simulink model "complex_with_subsystems"  (Simulink 8.0)
settings: Solver=ode45  StartTime=0.0  StopTime=10.0  MaxStep=0.1  RelTol=1e-3
settings Model: Creator=rstarr  LastModifiedBy=rstarr

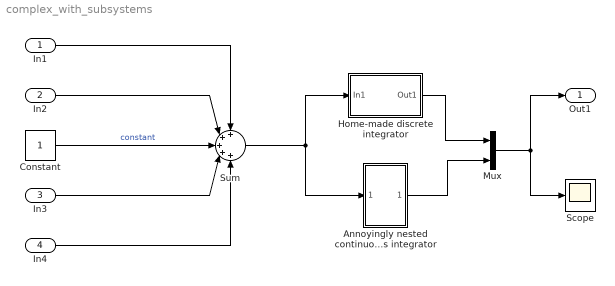
== system complex_with_subsystems ==
  In1 : Inport
  In2 : Inport  Port=2
  In3 : Inport  Port=3
  In4 : Inport  Port=4
  Annoyingly nested continuous integrator : Subsystem
  Constant : Constant
  Home-made discrete integrator : Subsystem
  Mux : Mux  Inputs=2
  Scope : Scope
  Sum : Sum  Inputs=+++++
  Out1 : Outport
  wires:
  Constant/1 -> Sum/3  "constant"
  In2/1 -> Sum/2
  In3/1 -> Sum/4
  In1/1 -> Sum/1
  In4/1 -> Sum/5
  Sum/1 -> Annoyingly nested continuous integrator/1(In1), Home-made discrete integrator/1(In1)
  Mux/1 -> Out1/1, Scope/1
  Home-made discrete integrator/1(Out1) -> Mux/1
  Annoyingly nested continuous integrator/1(Out1) -> Mux/2

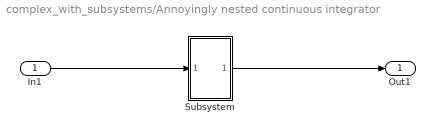
== system complex_with_subsystems/Annoyingly nested continuous integrator ==
  In1 : Inport
  Subsystem : Subsystem
  Out1 : Outport
  wires:
  In1/1 -> Subsystem/1(In1)
  Subsystem/1(Out1) -> Out1/1

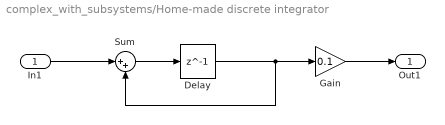
== system complex_with_subsystems/Home-made discrete integrator ==
  In1 : Inport
  Delay : Delay  DelayLength=1  InitialCondition=0  SampleTime=0.1
  Gain : Gain  Gain=0.1
  Sum : Sum  Inputs=|++
  Out1 : Outport
  wires:
  Delay/1 -> Sum/2, Gain/1
  Gain/1 -> Out1/1
  In1/1 -> Sum/1
  Sum/1 -> Delay/1

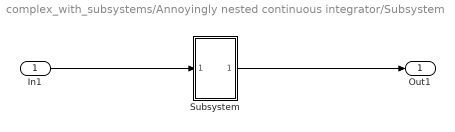
== system complex_with_subsystems/Annoyingly nested continuous integrator/Subsystem ==
  In1 : Inport
  Subsystem : Subsystem
  Out1 : Outport
  wires:
  In1/1 -> Subsystem/1(In1)
  Subsystem/1(Out1) -> Out1/1

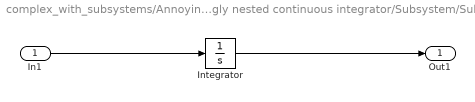
== system complex_with_subsystems/Annoyingly nested continuous integrator/Subsystem/Subsystem ==
  In1 : Inport
  Integrator : Integrator
  Out1 : Outport
  wires:
  In1/1 -> Integrator/1
  Integrator/1 -> Out1/1
